simulink model "Subsystem_StraightRoad_Challenge"  (R2023b)
settings: Solver=FixedStepDiscrete  StartTime=0.0  StopTime=10.0  RelTol=1e-3
model workspace (MAT data in the model file):
  firstWarning = 1
  originalScenarioChecksum = '01AEE5C4D9CCF9BA172694B67A97160A'
undefined symbols (not defined in the file): driving
libraries: drivingscenarioandsensors x10, sensorinslib x1
(part 1 of 4)
settings Model: Creator=victor  LastModifiedBy=victor

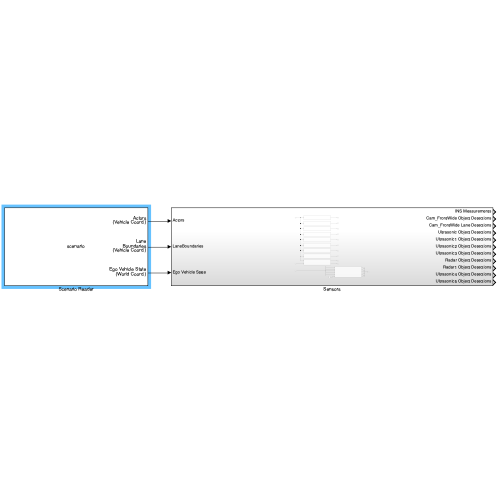
[thumbnail: Simulink's stored preview of the top-level diagram]
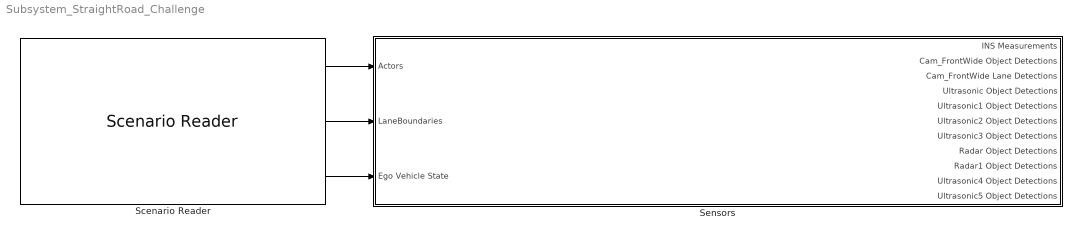
== system Subsystem_StraightRoad_Challenge ==
  Scenario Reader : drivingscenarioandsensors/Scenario Reader  ScenarioSource=From workspace  ScenarioFileName=/Users/victor/Documents/Duke/IndependentStudy/project/RNNMPC/Scenarios/StraightRoad_Challenge.mat  ScenarioVariableName=scenario  OutputCoordinateSystem=Vehicle coordinates  EgoVehicleSource=Scenario  EgoVehicleActorID=1  OrientVehiclesOnRoad=off  OutputEgoVehiclePose=off  OutputEgoVehicleState=on  SampleTime=0.1  LaneBoundaryOutput=Ego vehicle lane boundaries  LaneBoundaryDistance=linspace(-60, 60, 101)  LaneBoundaryLocation=Center of lane markings  BusNameSource=Auto  BusName=BusActors  BusNumActorsSource=Scenario  BusNumActors=100  BusName2Source=Auto  BusName2=BusLaneBoundaries  BusNumLaneBoundariesSource=Scenario  BusNumLaneBoundaries=10  BusName3Source=Auto  BusName3=BusEgoActor  BusName4Source=Auto  BusName4=BusEgoState  ShowCoordinateLabels=on  SimulateUsing=Interpreted execution
  Sensors : Subsystem
  wires:
  Scenario Reader/3 -> Sensors/3(Ego Vehicle State)
  Scenario Reader/2 -> Sensors/2(LaneBoundaries)
  Scenario Reader/1 -> Sensors/1(Actors)
